simulink model "lorenz4"  (Simulink 7.2)
settings: Solver=FixedStepDiscrete  StartTime=0.0  StopTime=1000  MaxStep=1  RelTol=1e-3
libraries: simulink x2, sldvlib x1
settings Model: Creator=nardi  LastModifiedBy=PauloAugusto  CovMetricSettings=dcmtrw  CovModelRefEnable=off
settings ConfigComp: Description=Design Verifier Custom Configuration Component  DVMode=PropertyProving  DVMaxProcessTime=600  DVDisplayUnsatisfiableObjectives=on  DVModelCoverageObjectives=MCDC  DVMaxTestCaseSteps=500  DVTestSuiteOptimization=CombinedObjectives  DVSaveHarnessModel=on  DVSaveReport=on

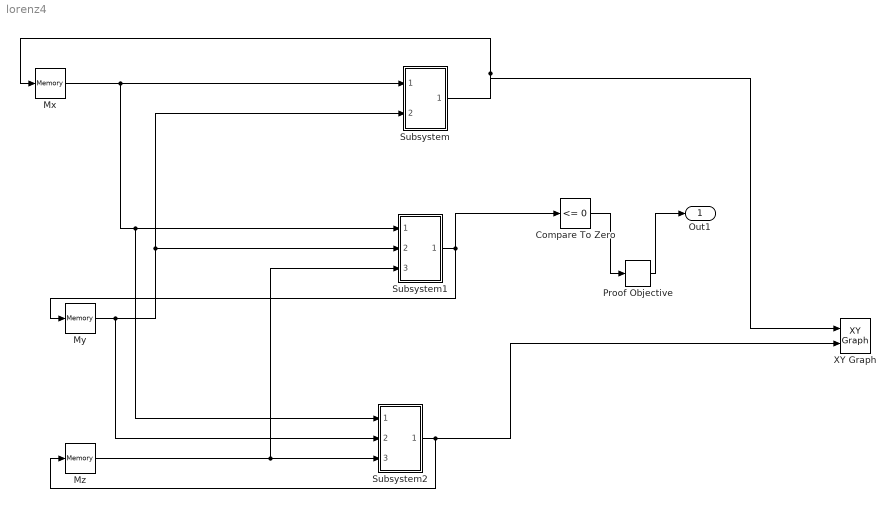
== system lorenz4 ==
  Compare To Zero : simulink/Logic and Bit Operations/Compare To Zero  SystemSampleTime=-1  relop=<=  LogicOutDataTypeMode=uint8  ZeroCross=off
  Mx : Memory
  My : Memory  X0=20
  Mz : Memory  X0=25
  Proof Objective : sldvlib/Proof Objective  SystemSampleTime=-1  enabled=on  customAVTBlockType=Proof Objective  intervals=0  dispValues=on  outEnabled=on
      settings: AttributesFormatString=%<intervals>
  Subsystem : Subsystem
  Subsystem1 : Subsystem
  Subsystem2 : Subsystem
  XY Graph : simulink/Sinks/XY Graph  SystemSampleTime=-1  xmin=-25  xmax=30  ymin=0  ymax=50  st=-1
  Out1 : Outport  OutDataType=sfix(16)  OutScaling=2^0
  wires:
  Mx/1 -> Subsystem/1(In1), Subsystem1/1(In1), Subsystem2/1(In1)
  My/1 -> Subsystem/2(In3), Subsystem1/2(In2), Subsystem2/2(In2)
  Subsystem/1(Out1) -> Mx/1, XY Graph/1
  Mz/1 -> Subsystem2/3(In3), Subsystem1/3(In3)
  Subsystem1/1(Out1) -> Compare To Zero/1, My/1
  Subsystem2/1(Out1) -> Mz/1, XY Graph/2
  Compare To Zero/1 -> Proof Objective/1
  Proof Objective/1 -> Out1/1

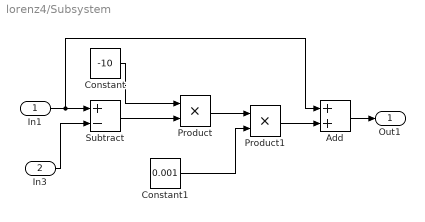
== system lorenz4/Subsystem ==
  In1 : Inport
  In3 : Inport  Port=2
  Add : Sum  OutDataType=sfix(16)  OutScaling=2^-10
  Constant : Constant  Value=-10  OutDataType=sfix(16)  OutScaling=2^0
  Constant1 : Constant  Value=0.001  OutDataType=sfix(16)  OutScaling=2^0
  Product : Product  OutDataType=sfix(16)  OutScaling=2^0  RndMeth=Zero
  Product1 : Product  OutDataType=sfix(16)  OutScaling=2^0  RndMeth=Zero
  Subtract : Sum  Inputs=+-  OutDataType=sfix(16)  OutScaling=2^-10
  Out1 : Outport  DataType=double  OutDataTypeStr=double
  wires:
  Product1/1 -> Add/2
  Constant1/1 -> Product1/2
  Product/1 -> Product1/1
  Constant/1 -> Product/1
  Subtract/1 -> Product/2
  In1/1 -> Subtract/1, Add/1
  In3/1 -> Subtract/2
  Add/1 -> Out1/1

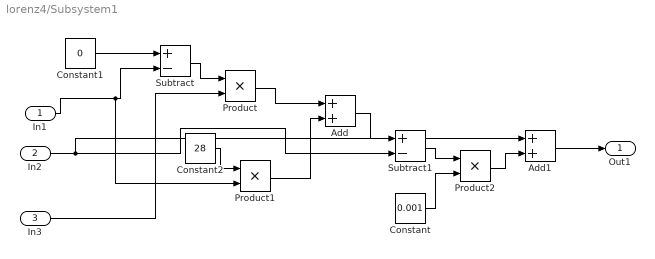
== system lorenz4/Subsystem1 ==
  In1 : Inport  OutDataType=sfix(16)  OutScaling=2^0
  In2 : Inport  Port=2  OutDataType=sfix(16)  OutScaling=2^0
  In3 : Inport  Port=3  OutDataType=sfix(16)  OutScaling=2^0
  Add : Sum  OutDataType=sfix(16)  OutScaling=2^-10
  Add1 : Sum  OutDataType=sfix(16)  OutScaling=2^-10
  Constant : Constant  Value=0.001  OutDataType=sfix(16)  OutScaling=2^0
  Constant1 : Constant  Value=0  OutDataType=sfix(16)  OutScaling=2^0
  Constant2 : Constant  Value=28  OutDataType=sfix(16)  OutScaling=2^0
  Product : Product  OutDataType=sfix(16)  OutScaling=2^0  RndMeth=Zero
  Product1 : Product  OutDataType=sfix(16)  OutScaling=2^0  RndMeth=Zero
  Product2 : Product  OutDataTypeMode=single  OutDataType=sfix(16)  OutScaling=2^0  OutDataTypeStr=single  RndMeth=Zero
  Subtract : Sum  Inputs=+-  OutDataType=sfix(16)  OutScaling=2^-10
  Subtract1 : Sum  Inputs=+-  OutDataType=sfix(16)  OutScaling=2^-10
  Out1 : Outport  DataType=double  OutDataType=sfix(16)  OutScaling=2^0  OutDataTypeStr=double
  wires:
  Constant1/1 -> Subtract/1
  In1/1 -> Subtract/2, Product1/2
  Subtract/1 -> Product/1
  In3/1 -> Product/2
  Product/1 -> Add/1
  Constant2/1 -> Product1/1
  In2/1 -> Subtract1/2, Add1/1
  Product1/1 -> Add/2
  Add/1 -> Subtract1/1
  Subtract1/1 -> Product2/1
  Constant/1 -> Product2/2
  Product2/1 -> Add1/2
  Add1/1 -> Out1/1

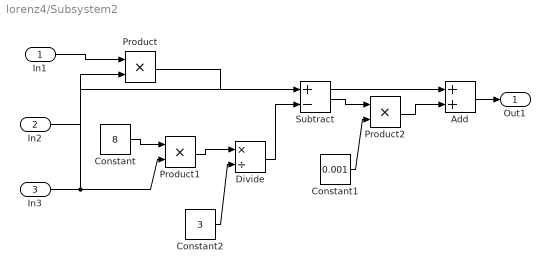
== system lorenz4/Subsystem2 ==
  In1 : Inport  OutDataType=sfix(16)  OutScaling=2^0
  In2 : Inport  Port=2  OutDataType=sfix(16)  OutScaling=2^0
  In3 : Inport  Port=3  OutDataType=sfix(16)  OutScaling=2^0
  Add : Sum  OutDataType=sfix(16)  OutScaling=2^-10
  Constant : Constant  Value=8  OutDataType=sfix(16)  OutScaling=2^0
  Constant1 : Constant  Value=0.001  OutDataType=sfix(16)  OutScaling=2^0
  Constant2 : Constant  Value=3  OutDataType=sfix(16)  OutScaling=2^0
  Divide : Product  Inputs=*/  OutDataType=sfix(16)  OutScaling=2^-10
  Product : Product  OutDataType=sfix(16)  OutScaling=2^0  RndMeth=Zero
  Product1 : Product  OutDataType=sfix(16)  OutScaling=2^0  RndMeth=Zero
  Product2 : Product  OutDataType=sfix(16)  OutScaling=2^0  RndMeth=Zero
  Subtract : Sum  Inputs=+-  OutDataType=sfix(16)  OutScaling=2^-10
  Out1 : Outport  DataType=double  OutDataType=sfix(16)  OutScaling=2^0  OutDataTypeStr=double
  wires:
  In1/1 -> Product/1
  In2/1 -> Product/2
  Constant/1 -> Product1/1
  In3/1 -> Product1/2, Add/1
  Product1/1 -> Divide/1
  Constant2/1 -> Divide/2
  Product/1 -> Subtract/1
  Divide/1 -> Subtract/2
  Subtract/1 -> Product2/1
  Constant1/1 -> Product2/2
  Product2/1 -> Add/2
  Add/1 -> Out1/1
